simulink model "Capacitor_system"  (R2024b)
settings: Solver=VariableStepAuto  StartTime=0.0  StopTime=10.0  RelTol=1e-3
model workspace (MAT data in the model file):
  C = 1e-06
settings Model: Creator=omari  LastModifiedBy=omari

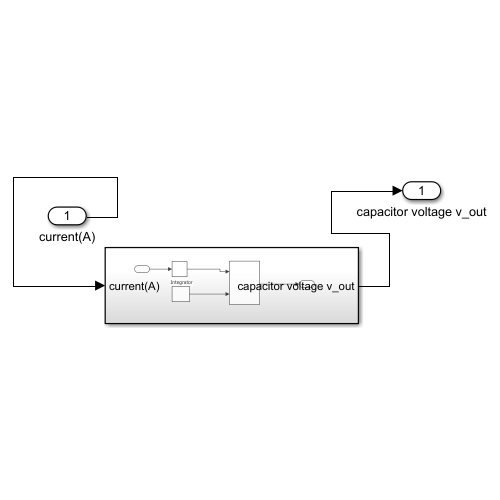
[thumbnail: Simulink's stored preview of the top-level diagram]
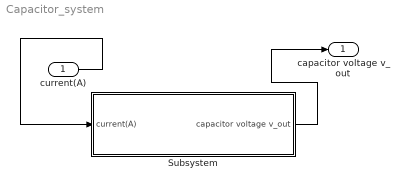
== system Capacitor_system ==
  current(A) : Inport
  Subsystem : Subsystem
  capacitor voltage v_out : Outport
  wires:
  current(A)/1 -> Subsystem/1(current(A))
  Subsystem/1(capacitor voltage v_out) -> capacitor voltage v_out/1

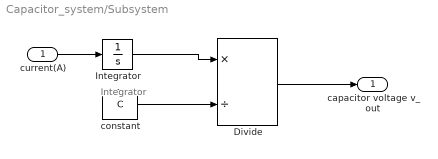
== system Capacitor_system/Subsystem ==
  note: Integrator
  current(A) : Inport
  Divide : Product  Inputs=*/
  Integrator : Integrator
  constant : Constant  Value=C
  capacitor voltage v_out : Outport
  wires:
  Integrator/1 -> Divide/1
  current(A)/1 -> Integrator/1
  constant/1 -> Divide/2
  Divide/1 -> capacitor voltage v_out/1
